simulink model "Controller"  (R2018b)
settings: Solver=VariableStepAuto  StartTime=0.0  StopTime=10.0  RelTol=1e-3
libraries: mpclib x1
settings Model: Creator=Yahya  LastModifiedBy=Yahya

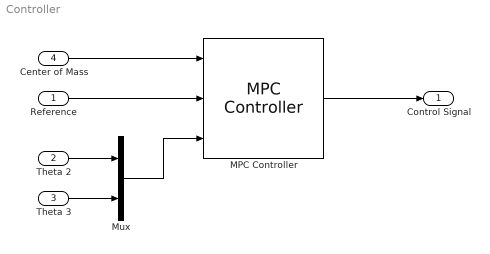
== system Controller ==
  Reference : Inport
  Theta 2 : Inport  Port=2
  Theta 3 : Inport  Port=3
  Center of Mass : Inport  Port=4
  MPC Controller : mpclib/MPC Controller  SCDEnableBlockLinearizationSpecification=on  is_multiple=0  enable_value=0  return_u0=off  updateMPCinCallerWorkspace=on  md_inport=on  mv_inport=off  return_cost=off  return_mvseq=off  return_qpstatus=off  return_xseq=off  return_state=off  return_ovseq=off  state_inport=off  umin_inport=off  umax_inport=off  ymin_inport=off  ymax_inport=off  cc_inport=off  ywt_inport=off  uwt_inport=off  duwt_inport=off  rhoeps_inport=off  uref_inport=off  n_ts=0.1  n_p=10  n_mv=1  n_md=2  n_ud=0  n_mo=1  n_uo=0  BlockDataType=double  SampleTimeInherited=off  switch_inport=off
  Mux : Mux  Inputs=2
  Control Signal : Outport
  wires:
  Center of Mass/1 -> MPC Controller/1
  Reference/1 -> MPC Controller/2
  MPC Controller/1 -> Control Signal/1
  Mux/1 -> MPC Controller/3
  Theta 2/1 -> Mux/1
  Theta 3/1 -> Mux/2
